simulink model "mdl_GPSreceiveBin1"  (R2020b)
settings: Solver=FixedStepDiscrete  StartTime=0.0  StopTime=10.0  RelTol=1e-3  EnableMultiTasking=on
undefined symbols (not defined in the file): Green, led0
libraries: raspberrypiBasiclib x1, raspberrypiCommlib x1
settings Model: ModifiedByFormat=The MathWorks Inc.  SimulationMode=external  EnablePacing=on  Creator=The MathWorks, Inc.  LastModifiedBy=The MathWorks Inc.
settings SolverCC: PositivePriorityOrder=on
settings DataIOCC: LimitDataPoints=on  SaveFormat=Array  ReturnWorkspaceOutputs=off
settings OptimizationCC: LifeSpan=1  MaxStackSize=64
settings DebuggingCC: UnderspecifiedInitializationDetection=Classic  MergeDetectMultiDrivingBlocksExec=none  SolverPrmCheckMsg=warning  AllowSymbolicDim=off  SFUnexpectedBacktrackingDiag=warning  SFNoUnconditionalDefaultTransitionDiag=warning  SFExecutionAtInitializationDiag=none  ArithmeticOperatorsInVariantConditions=warning
settings HardwareCC: ProdBitPerPointer=32  ProdBitPerSizeT=32  ProdBitPerPtrDiffT=32  ProdLargestAtomicInteger=Long  ProdLargestAtomicFloat=Double  ProdWordSize=32  ProdHWDeviceType=ARM Compatible->ARM Cortex  UseEmbeddedCoderFeatures=off  UseSimulinkCoderFeatures=off
settings ModelReferenceCC: PropagateSignalLabelsOutOfModel=off
settings SFSimCC: SimUseLocalCustomCode=off  MATLABDynamicMemAlloc=off  CustomCodeUndefinedFunction=UseInterfaceOnly
settings RTWCC: Description=Embedded Coder  SystemTargetFile=ert.tlc  HardwareBoard=Raspberry Pi  TemplateMakefile=ert_default_tmf  RTWUseLocalCustomCode=off  Toolchain=GNU GCC Raspberry Pi
settings CodeAppCC: StateflowObjectComments=on
settings ERTTargetCC: MultiwordLength=2048  ERTCustomFileBanners=off  SupportContinuousTime=on  SupportNonInlinedSFcns=on  RemoveResetFunc=off  ModelStepFunctionPrototypeControlCompliant=off  ConvertIfToSwitch=off  SuppressUnreachableDefaultCases=off
settings ConfigComp: CovMetricSettings=dw  CovSaveCumulativeToWorkspaceVar=on  CovSaveSingleToWorkspaceVar=on  CovExternalEMLEnable=off  CovSFcnEnable=off

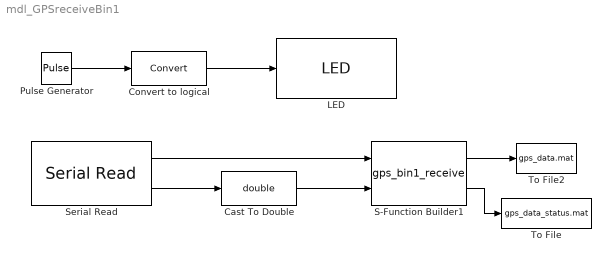
== system mdl_GPSreceiveBin1 ==
  Cast To Double : DataTypeConversion  OutDataTypeStr=double
  Convert to logical : DataTypeConversion
  LED : raspberrypiBasiclib/LED  BoardProperty=Pi 4 Model B  LED_=led0 (Green)
      settings: SourceProductName=Simulink Support Package for Raspberry Pi Hardware
  Pulse Generator : DiscretePulseGenerator  Period=10  PulseWidth=5  SampleTime=0.1
  S-Function Builder1 : S-Function  FunctionName=gps_bin1_receive  SFunctionModules=gps_bin1_receive_wrapper  SFunctionDeploymentMode=off  EnableBusSupport=off  mask(S-Function Builder){}
      mask help: Simulink:masks:SFunctionBuilder_MD
      mask init:
      | val = [[.9  0.75 0.75 1 1 .9 .9 1]',[1 1 0.75 0.75 .9 .9 1 .9]'];try , sys = get_param(gcb,'SfunBuilderFcnName');if isempty(sys), sys = get_param(gcb,'FunctionName'); end,catch, sys = get_param(gcb,'FunctionName'); end
      settings: CopyFcn=set_param(gcbh,'LinkStatus','none')  OpenFcn=sfunctionwizard(gcbh)
      mask Display: plot(val(:,1),val(:,2)),disp(sys),port_label('input',1,'u0'),port_label('input',2,'u1'),port_label('output',1,'y0'),port_label('output',2,'y1')
  Serial Read : raspberrypiCommlib/Serial Read  board=Pi 4 Model B  SCIModule_=/dev/serial0  Baudrate_=19200  Parity=None  StopBits_=1  HardwareFlowControl=None  ByteOrder=LittleEndian  DataLength=64  DataType=uint8  OutputStatus=on  SampleTime=0.1  blockPlatform=RaspberryPi
      settings: SourceProductBaseCode=RASPPI
  To File : ToFile  Filename=gps_data_status.mat
  To File2 : ToFile  Filename=gps_data.mat
  wires:
  Pulse Generator/1 -> Convert to logical/1
  Convert to logical/1 -> LED/1
  Serial Read/1 -> S-Function Builder1/1
  S-Function Builder1/2 -> To File/1
  Serial Read/2 -> Cast To Double/1
  S-Function Builder1/1 -> To File2/1
  Cast To Double/1 -> S-Function Builder1/2
